simulink model "Ex01_eval"  (R2020a)
settings: Solver=VariableStepAuto  StartTime=0.0  StopTime=50  RelTol=1e-3
values from neighbouring files (symbols this model uses):
  FLAG = 1    [evalGamma.m]
settings Model: Creator=FawaD KhaN  LastModifiedBy=Zeeshan Iqbal Khan

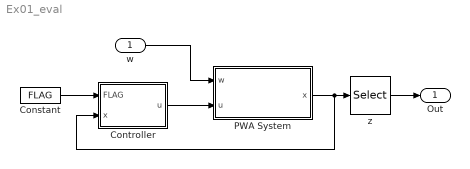
== system Ex01_eval ==
  w : Inport
  Constant : Constant  Value=FLAG
  Controller : MATLAB Function  TreatAsAtomicUnit=on
  PWA System : Subsystem
  z : Selector  InputPortWidth=5  IndexOptions=Index vector (dialog)  Indices=[1]  OutputSizes=1
  Out : Outport
  wires:
  PWA System/1(x) -> z/1, Controller/2(x)
  Controller/1(u) -> PWA System/2(u)
  Constant/1 -> Controller/1(FLAG)
  w/1 -> PWA System/1(w)
  z/1 -> Out/1

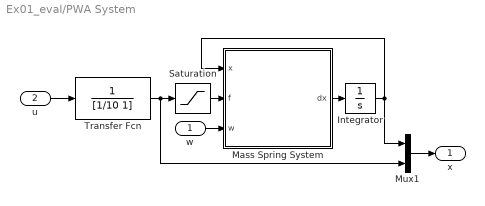
== system Ex01_eval/PWA System ==
  w : Inport
  u : Inport  Port=2
  Integrator : Integrator  InitialCondition=[5;-5;0;0]
  Mass Spring System : MATLAB Function  TreatAsAtomicUnit=on
  Mux1 : Mux  Inputs=2
  Saturation : Saturate  UpperLimit=1  LowerLimit=-1
  Transfer Fcn : TransferFcn  Denominator=[1/10 1]
  x : Outport
  wires:
  u/1 -> Transfer Fcn/1
  Transfer Fcn/1 -> Saturation/1, Mux1/2
  Saturation/1 -> Mass Spring System/2(f)
  Integrator/1 -> Mux1/1, Mass Spring System/1(x)
  Mass Spring System/1(dx) -> Integrator/1
  Mux1/1 -> x/1
  w/1 -> Mass Spring System/3(w)

== matlab function Ex01_eval/PWA System/Mass Spring System ==
  data: x input; f input; w input; dx output
function dx = fcn(x,f,w)

M1 = 1;   M2 = 1;
k1 = 1;   k2 = 1;
b1 = 0.1; b2 = 0.1;

M = blkdiag(M1,M2);

C = [b1+b2, -b2;
       -b1,  b2];

K = [k1+k2, -k2;
       -k1,  k2];
A0 = [zeros(2), eye(2); -M\K, -M\C];
B0 = [zeros(2); M\eye(2)];


% dx = zeros(4,1);
dx = A0*x(:) + B0*[w;f];

% dx(1,1) = x(3);
% dx(2,1) = x(4);
% dx(3,1) = (-(k1+k2)*x(1) - (b1+b2)*x(2) + k2*x(3) + b2*x(4) + w)/M1;
% dx(4,1) = (k2*x(1) + b2*x(2) - k2*x(3) - b2*x(4) + u)/M2;
end

== matlab function Ex01_eval/Controller ==
  data: FLAG input; x input; u output
function u  = fcn(FLAG,x)
if(FLAG == 0)
    if x(5) < -1
        K = [0.16481 -0.042629 -3.0148 -5.2692 -0.37877];
    elseif x(5) > 1
        K  = [0.16481 -0.042629 -3.0148 -5.2692 -0.37877];
    else
        K  = [0.42911 -0.56227 -10.943 -19.029 -3.591];
    end
else
    K = [2.45 -12.50 -401.3 -645.3 -172.0];
end
u = K*x;
end
